simulink model "es2_sim"  (R2023b)
settings: Solver=VariableStepAuto  StartTime=0.0  StopTime=10.0  RelTol=1e-3
values from neighbouring files (symbols this model uses):
  Alin = J1    [es2.m]
  Blin = double(jacobian(f,u))    [es2.m]
  Clin = double(jacobian(y, [x1 x2]))    [es2.m]
  ueq = 0.5    [es2.m]
  x0 = [0.1;6]    [es2.m]
  xeq1 = double([xeq_s.x1(1) xeq_s.x2(1)])    [es2.m]
settings Model: Creator=stefa  LastModifiedBy=stefa

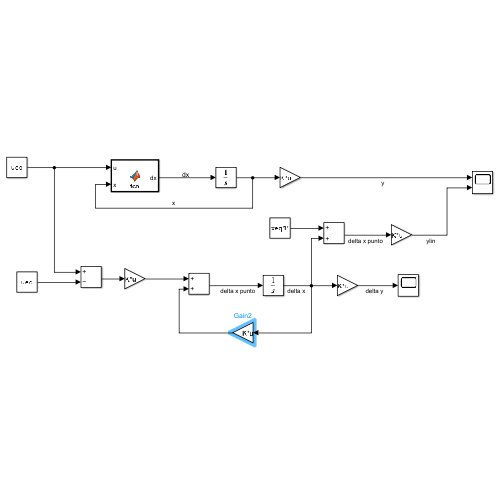
[thumbnail: Simulink's stored preview of the top-level diagram]
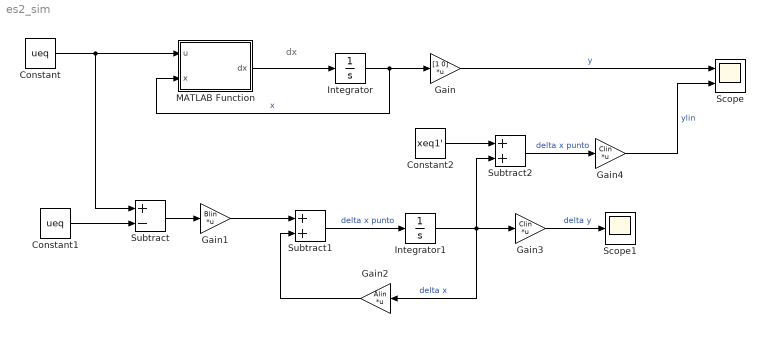
== system es2_sim ==
  note: dx
  Constant : Constant  Value=ueq
  Constant1 : Constant  Value=ueq
  Constant2 : Constant  Value=xeq1'
  Gain : Gain  Gain=[1 0]  Multiplication=Matrix(K*u)
  Gain1 : Gain  Gain=Blin  Multiplication=Matrix(K*u)
  Gain2 : Gain  Gain=Alin  Multiplication=Matrix(K*u)
  Gain3 : Gain  Gain=Clin  Multiplication=Matrix(K*u)
  Gain4 : Gain  Gain=Clin  Multiplication=Matrix(K*u)
  Integrator : Integrator  InitialCondition=x0
  Integrator1 : Integrator  InitialCondition=x0-xeq1'
  MATLAB Function : MATLAB Function  TreatAsAtomicUnit=on
  Scope : Scope  NumInputPorts=2
  Scope1 : Scope
  Subtract : Sum  Inputs=+-
  Subtract1 : Sum
  Subtract2 : Sum
  wires:
  MATLAB Function/1(dx) -> Integrator/1
  Integrator/1 -> Gain/1, MATLAB Function/2(x)  "x"
  Gain/1 -> Scope/1  "y"
  Constant/1 -> Subtract/1, MATLAB Function/1(u)
  Subtract/1 -> Gain1/1
  Integrator1/1 -> Gain2/1, Subtract2/2, Gain3/1  "delta x"
  Gain2/1 -> Subtract1/2
  Subtract1/1 -> Integrator1/1  "delta x punto"
  Gain1/1 -> Subtract1/1
  Gain3/1 -> Scope1/1  "delta y"
  Constant1/1 -> Subtract/2
  Constant2/1 -> Subtract2/1
  Subtract2/1 -> Gain4/1  "delta x punto"
  Gain4/1 -> Scope/2  "ylin"

== matlab function es2_sim/MATLAB Function ==
  data: u input; dx output; x input
function dx = fcn(u,x)

x1=x(1);
x2=x(2);

dx = [x1*(0.01*x1-1)+(x1*x2)/50;0.001*(x1*x2)/1000-0.1*x2+u];
